simulink model "matlab"  (R2023b)
settings: Solver=ode15s  StartTime=0.0  StopTime=0.25  MaxStep=1e-6  RelTol=1e-4  EnableMultiTasking=on
libraries: spsSeriesRLCBranchLib x6, spsDiodeLib x3, spsCurrentMeasurementLib x2, spsMosfetLib x2, simulink x2, spsVoltageMeasurementLib x2, spsControlledVoltageSourceLib x1, spsMeanLib x1, spspowerguiLib x1
settings Model: Creator=cse  LastModifiedBy=Krish
settings SolverCC: AlgebraicLoopSolver=TrustRegion
settings DataIOCC: LimitDataPoints=on  SaveFormat=Array  ReturnWorkspaceOutputs=off
settings OptimizationCC: LifeSpan=inf
settings DebuggingCC: UnderspecifiedInitializationDetection=Classic  MergeDetectMultiDrivingBlocksExec=none  SolverPrmCheckMsg=warning  UnconnectedInputMsg=warning  UnconnectedOutputMsg=warning  UnconnectedLineMsg=warning  StateNameClashWarn=warning  SFUnexpectedBacktrackingDiag=warning  SFNoUnconditionalDefaultTransitionDiag=warning  SFExecutionAtInitializationDiag=none  ArithmeticOperatorsInVariantConditions=warning
settings HardwareCC: ProdBitPerPointer=32  ProdBitPerSizeT=32  ProdBitPerPtrDiffT=32  ProdLargestAtomicFloat=None  ProdIntDivRoundTo=Undefined  ProdEndianess=Unspecified  ProdWordSize=32  ProdHWDeviceType=32-bit Generic
settings ModelReferenceCC: EnableRefExpFcnMdlSchedulingChecks=on  PropagateSignalLabelsOutOfModel=off
settings SFSimCC: SimUseLocalCustomCode=off  CustomCodeUndefinedFunction=UseInterfaceOnly
settings RTWCC: RTWUseLocalCustomCode=off  DLArmComputeVersion=19.05
settings CodeAppCC: StateflowObjectComments=on
settings GRTTargetCC: TargetLangStandard=C89/C90 (ANSI)
settings ConfigComp: CovMetricSettings=dw  CovSaveCumulativeToWorkspaceVar=on  CovSaveSingleToWorkspaceVar=on  CovExternalEMLEnable=off
settings SimscapeCC: SimscapeNormalizeSystem=off

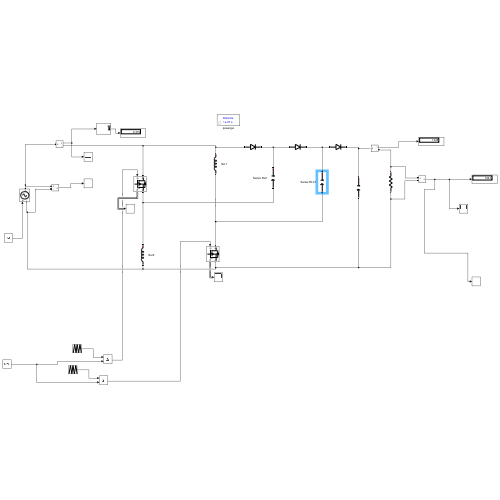
[thumbnail: Simulink's stored preview of the top-level diagram]
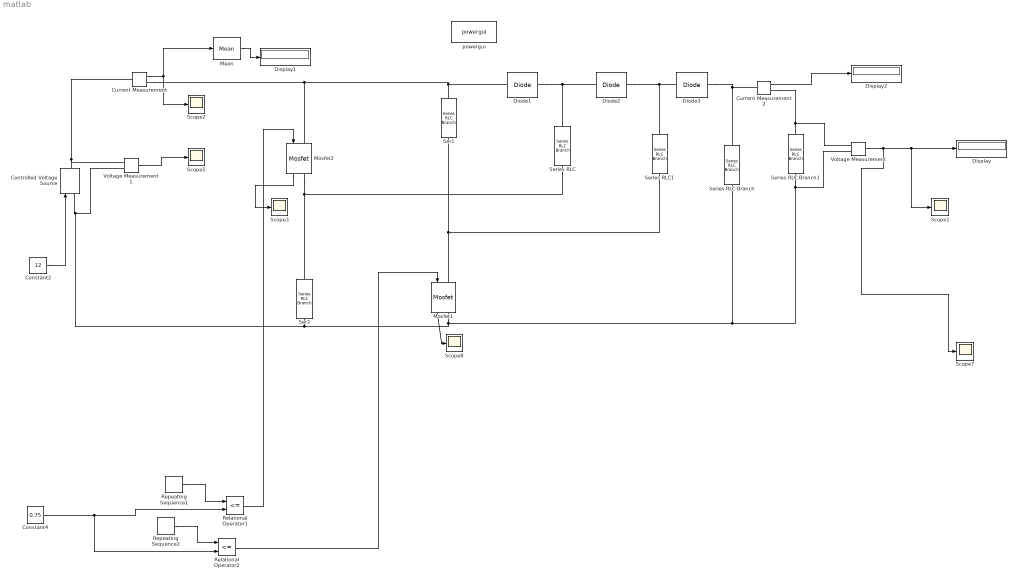
== system matlab ==
  Constant2 : Constant  Value=12
  Constant4 : Constant  Value=0.75
  Controlled Voltage Source : spsControlledVoltageSourceLib/Controlled Voltage Source  Initialize=on  Source_Type=AC  Amplitude=0  Phase=0  Frequency=0  Measurements=None
  Current Measurement : spsCurrentMeasurementLib/Current Measurement  PhasorSimulation=off  OutputType=Complex  PSBequivalent=0
  Current Measurement2 : spsCurrentMeasurementLib/Current Measurement  PhasorSimulation=off  OutputType=Complex  PSBequivalent=0
  Diode1 : spsDiodeLib/Diode  Ron=57e-3  Lon=0  Vf=0.57  IC=0  UseSnubber=off  Rs=inf  Cs=250e-9  Measurements=off
  Diode2 : spsDiodeLib/Diode  Ron=57e-3  Lon=0  Vf=0.57  IC=0  UseSnubber=off  Rs=inf  Cs=250e-9  Measurements=off
  Diode3 : spsDiodeLib/Diode  Ron=57e-3  Lon=0  Vf=0.57  IC=0  UseSnubber=off  Rs=inf  Cs=250e-9  Measurements=off
  Display : Display
  Display1 : Display
  Display2 : Display
  Mean : spsMeanLib/Mean  Freq=33000  Vinit=0  Ts=1e-6
  Mosfet1 : spsMosfetLib/Mosfet  Ron=9e-3  Lon=0  Rd=0.01  Vfd=0  IC=0  Rs=1e5  Cs=inf  Measurements=on
  Mosfet2 : spsMosfetLib/Mosfet  Ron=9e-3  Lon=0  Rd=0.01  Vfd=0  IC=0  Rs=1e5  Cs=inf  Measurements=on
  Relational Operator1 : RelationalOperator  Operator=<=  OutDataTypeStr=boolean  RndMeth=Simplest  InputSameDT=off
  Relational Operator2 : RelationalOperator  Operator=<=  OutDataTypeStr=boolean  RndMeth=Simplest  InputSameDT=off
  Repeating Sequence1 : simulink/Sources/Repeating Sequence  rep_seq_t=[0 0.5 1]/33000  rep_seq_y=[0 1 0]
  Repeating Sequence2 : simulink/Sources/Repeating Sequence  rep_seq_t=[0 0.5 1]/33000  rep_seq_y=[0 1 0]
  Scope{1..3,5,7..8} (6 alike) : Scope
  Ser1 : spsSeriesRLCBranchLib/Series RLC Branch  LConnTagsString=__new0  RConnTagsString=__new0  BranchType=L  Resistance=17e-3  Inductance=500e-6  SetiL0=off  InitialCurrent=0  Capacitance=1e-6  Setx0=off  InitialVoltage=0  Measurements=Branch current
  Ser2 : spsSeriesRLCBranchLib/Series RLC Branch  LConnTagsString=__new0  RConnTagsString=__new0  BranchType=L  Resistance=17e-3  Inductance=500e-6  SetiL0=off  InitialCurrent=0  Capacitance=1e-6  Setx0=off  InitialVoltage=0  Measurements=Branch current
  Series RLC : spsSeriesRLCBranchLib/Series RLC Branch  LConnTagsString=__new0  RConnTagsString=__new0  BranchType=C  Resistance=3e-3  Inductance=1e-3  SetiL0=off  InitialCurrent=0  Capacitance=50e-6  Setx0=off  InitialVoltage=0  Measurements=Branch voltage
  Series RLC Branch : spsSeriesRLCBranchLib/Series RLC Branch  LConnTagsString=__new0  RConnTagsString=__new0  BranchType=C  Resistance=3e-3  Inductance=1e-3  SetiL0=off  InitialCurrent=0  Capacitance=100e-6  Setx0=off  InitialVoltage=0  Measurements=None
  Series RLC Branch1 : spsSeriesRLCBranchLib/Series RLC Branch  LConnTagsString=__new0  RConnTagsString=__new0  BranchType=R  Resistance=100  Inductance=1e-3  SetiL0=off  InitialCurrent=0  Capacitance=1e-6  Setx0=off  InitialVoltage=0  Measurements=None
  Series RLC1 : spsSeriesRLCBranchLib/Series RLC Branch  LConnTagsString=__new0  RConnTagsString=__new0  BranchType=C  Resistance=3e-3  Inductance=1e-3  SetiL0=off  InitialCurrent=0  Capacitance=50e-6  Setx0=off  InitialVoltage=0  Measurements=Branch voltage
  Voltage Measurement : spsVoltageMeasurementLib/Voltage Measurement  PhasorSimulation=off  OutputType=Complex  PSBequivalent=0
  Voltage Measurement1 : spsVoltageMeasurementLib/Voltage Measurement  PhasorSimulation=off  OutputType=Complex  PSBequivalent=0
  powergui : spspowerguiLib/powergui  Priority=1  SimulationMode=Discrete  SampleTime=0.1e-6  frequency=60  Iterations=50  frequencyindice=0  Pbase=100e6  ErrMax=1e-4  UnitsV=kV  UnitsW=MW  buscounter=0  FunctionMessages=off  echomessages=off  EnableUseOfTLC=off  CurrentSourceSwitches=off  DisableSnubberDevices=off  DisableRonSwitches=off  DisableVfSwitches=off  DisplayEquations=off  AutomaticDiscreteSolvers=off  SolverType=Tustin/Backward Euler (TBE)  Interpol=off  ExternalGateDelay=off  methode=off  Ts=100  x0status=blocks  SPID=on  SwTol=0  HookPort=off  NonlinearTolerance=1e-4  nMaxIteration=100  ContinueOnMaxIteration=off  RestoreLinks=warning  ResistiveCurrentMeasurement=off  Frange=[0:2:500]  Ylog=off  Xlog=on  ShowGrid=off  save=off  variable=ZData  structure=0  ZoomFFT=off  StartTime=0.0  cycles=1  DisplayStyle=1  fundamental=60  FreqAxis=off  MaxFrequency=1000  frequencyindicesteady=1  RmsSteady=1  display=off
  wires:
  Current Measurement/1 -> Scope2/1, Mean/1
  Mean/1 -> Display1/1
  Voltage Measurement1/1 -> Scope5/1
  Voltage Measurement/1 -> Scope7/1, Scope1/1, Display/1
  Current Measurement2/1 -> Display2/1
  Constant2/1 -> Controlled Voltage Source/1
  Mosfet1/1 -> Scope8/1
  Mosfet2/1 -> Scope3/1
  Repeating Sequence1/1 -> Relational Operator1/1
  Repeating Sequence2/1 -> Relational Operator2/1
  Constant4/1 -> Relational Operator2/2, Relational Operator1/2
  Relational Operator1/1 -> Mosfet2/1
  Relational Operator2/1 -> Mosfet1/1
  connections:
  Current Measurement/LConn1 -- Voltage Measurement1/LConn1 -- Controlled Voltage Source/RConn1
  Mosfet2/RConn1 -- Series RLC/RConn1 -- Ser2/LConn1
  Current Measurement2/LConn1 -- Diode3/RConn1 -- Series RLC Branch/LConn1
  Series RLC Branch/RConn1 -- Voltage Measurement1/LConn2 -- Controlled Voltage Source/LConn1 -- Ser2/RConn1 -- Mosfet1/RConn1 -- Voltage Measurement/LConn2 -- Series RLC Branch1/RConn1
  Current Measurement2/RConn1 -- Series RLC Branch1/LConn1 -- Voltage Measurement/LConn1
  Mosfet1/LConn1 -- Series RLC1/RConn1 -- Ser1/RConn1
  Ser1/LConn1 -- Diode1/LConn1 -- Current Measurement/RConn1 -- Mosfet2/LConn1
  Diode2/RConn1 -- Series RLC1/LConn1 -- Diode3/LConn1
  Diode1/RConn1 -- Series RLC/LConn1 -- Diode2/LConn1
